simulink model "Totem_Pole_PFC_v1"  (R2024b)
settings: Solver=FixedStepDiscrete  StartTime=0.0  StopTime=0.6  FixedStep=Ts_Power  MaxStep=1e-7  RelTol=1e-4  EnableMultiTasking=on
PreLoadFcn:
  | Totem_Pole_PFC_v1_data
values from neighbouring files (symbols this model uses):
  C_PFC = 2600e-6    (= 0.0026)    [OBC_v1_data.m]    (also in Totem_Pole_PFC_v1_data.m)
  Fnom = 60    [OBC_v1_data.m]    (also in Totem_Pole_PFC_v1_data.m)
  Fr_I = Fnom*2    (= 120)    [OBC_v1_data.m]    (also in Totem_Pole_PFC_v1_data.m)
  Ki_V = 80    [OBC_v1_data.m]    (also in Totem_Pole_PFC_v1_data.m)
  Kp_I = 0.06    [OBC_v1_data.m]    (also in Totem_Pole_PFC_v1_data.m)
  Kp_V = 0.25    [OBC_v1_data.m]    (also in Totem_Pole_PFC_v1_data.m)
  Kr_I = 2.5    [OBC_v1_data.m]    (also in Totem_Pole_PFC_v1_data.m)
  L_PFC = 600e-6    (= 0.0006)    [OBC_v1_data.m]    (also in Totem_Pole_PFC_v1_data.m)
  Limit_V = 100    [OBC_v1_data.m]    (also in Totem_Pole_PFC_v1_data.m)
  RL_PFC = 20e-3    (= 0.02)    [OBC_v1_data.m]    (also in Totem_Pole_PFC_v1_data.m)
  Ro = Vo_nom^2/Po_nom    (= 22.2222222222)    [LLC_Resonant_Converter_v1_data.m]    (also in OBC_v1_data.m; Totem_Pole_PFC_v1_data.m = 22.22)
  Ts_Control = 10e-6    (= 1e-05)    [LLC_Resonant_Converter_v1_data.m]    (also in OBC_v1_data.m; Totem_Pole_PFC_v1_data.m)
  Ts_Power = 50e-9    (= 5e-08)    [LLC_Resonant_Converter_v1_data.m]    (also in OBC_v1_data.m; Totem_Pole_PFC_v1_data.m)
  Vnom_ac = 240    [OBC_v1_data.m]    (also in Totem_Pole_PFC_v1_data.m)
undefined symbols (not defined in the file or in its folder): DiscIntNeverNeededParam
libraries: spsSeriesRLCBranchLib x4, spsDiodeLib x3, spsMeanLib x3, spsCurrentMeasurementLib x2, MyLibrary x2, spsFourierLib x2, simulink x2, spsVoltageMeasurementLib x2, spsACVoltageSourceLib x1, spsIdealSwitchLib x1, spsPowerLib x1, spsTHDLib x1
settings Model: SimulationMode=accelerator  Creator=The MathWorks, Inc.  LastModifiedBy=santh
settings SolverCC: AlgebraicLoopSolver=TrustRegion  SolverResetMethod=Robust
settings DataIOCC: SaveOutput=off  SignalLogging=off  DSMLogging=off  SaveTime=off  ReturnWorkspaceOutputs=off
settings OptimizationCC: LifeSpan=inf
settings DebuggingCC: UnconnectedInputMsg=warning  UnconnectedOutputMsg=warning  UnconnectedLineMsg=warning  SFUnexpectedBacktrackingDiag=warning  SFNoUnconditionalDefaultTransitionDiag=warning  SFExecutionAtInitializationDiag=none  ArithmeticOperatorsInVariantConditions=warning
settings ModelReferenceCC: EnableRefExpFcnMdlSchedulingChecks=on
settings SFSimCC: SimUseLocalCustomCode=off  CustomCodeUndefinedFunction=UseInterfaceOnly
settings RTWCC: RTWUseLocalCustomCode=off  GPUComputeCapability=3.5  DLArmComputeVersion=19.05
settings CodeAppCC: StateflowObjectComments=on
settings GRTTargetCC: TargetLangStandard=C89/C90 (ANSI)
settings ConfigComp: CovMetricSettings=dw  CovSaveCumulativeToWorkspaceVar=on  CovSaveSingleToWorkspaceVar=on  CovExternalEMLEnable=off
settings SimscapeCC: SimscapeNormalizeSystem=off  SimscapeNominalValues={1, 'bar'; 1, 'cm^3/s'; 1, 'bar*kg/s'; 1, 'kJ/kg'; 1, 'kW'; }

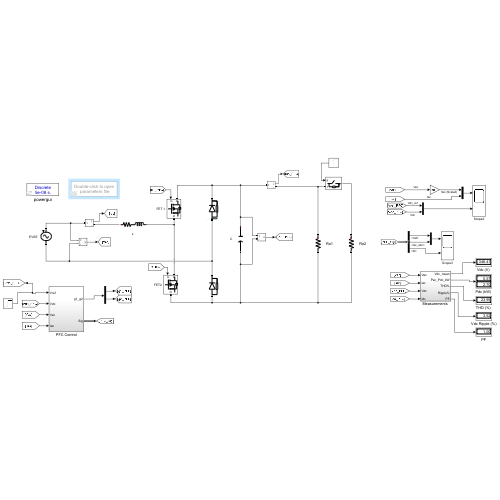
[thumbnail: Simulink's stored preview of the top-level diagram]
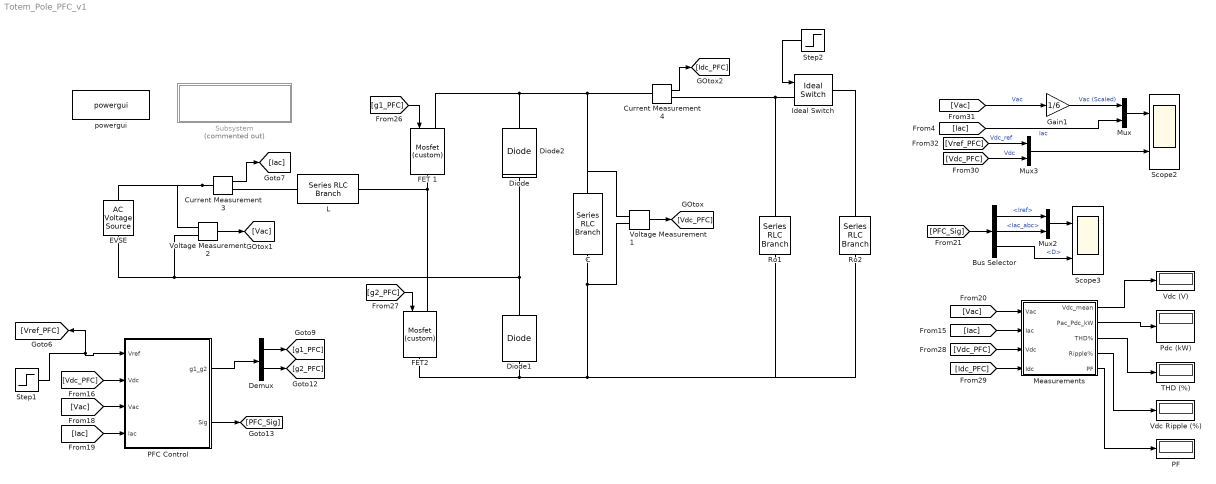
== system Totem_Pole_PFC_v1 ==
  Bus Selector : BusSelector  OutputSignals=Iref,Iac_abc,D
  C : spsSeriesRLCBranchLib/Series RLC Branch  LConnTagsString=__new0  RConnTagsString=__new0  BranchType=C  Resistance=1  Inductance=1e-3  SetiL0=off  InitialCurrent=0  Capacitance=C_PFC  Setx0=on  InitialVoltage=375  Measurements=None
  Current Measurement3 : spsCurrentMeasurementLib/Current Measurement  PhasorSimulation=off  OutputType=Complex  PSBequivalent=0
  Current Measurement4 : spsCurrentMeasurementLib/Current Measurement  PhasorSimulation=off  OutputType=Complex  PSBequivalent=0
  Demux : Demux  Outputs=2
  Diode : spsDiodeLib/Diode  Ron=Ron_Diode  Lon=0  Vf=Vf  IC=0  UseSnubber=0  Rs=1e6  Cs=inf  Measurements=off
  Diode1 : spsDiodeLib/Diode  Ron=Ron_Diode  Lon=0  Vf=Vf  IC=0  UseSnubber=0  Rs=1e6  Cs=inf  Measurements=off
  Diode2 : spsDiodeLib/Diode  Ron=Ron_Diode  Lon=0  Vf=Vf  IC=0  UseSnubber=0  Rs=1e6  Cs=inf  Measurements=off
  EVSE : spsACVoltageSourceLib/AC Voltage Source  Amplitude=Vnom_ac*sqrt(2)  Phase=0  Frequency=Fnom  SampleTime=Ts_Power  Measurements=None  BusType=swing  Pref=10e3  Qref=0  Qmin=-inf  Qmax=+inf
  FET 1 : MyLibrary/Mosfet (custom)  Ron=Ron_FET  Lon=0  Rd=Ron_Diode  Vfd=Vf  IC=0  Rs=1e6  Cs=inf  Measurements=off
  FET2 : MyLibrary/Mosfet (custom)  Ron=Ron_FET  Lon=0  Rd=Ron_Diode  Vfd=Vf  IC=0  Rs=1e6  Cs=inf  Measurements=off
  Gain1 : Gain  Gain=1/6
  Ideal Switch : spsIdealSwitchLib/Ideal Switch  Ron=0.001  Lon=0  IC=0  Rs=1e5  Cs=inf  Measurements=off
  L : spsSeriesRLCBranchLib/Series RLC Branch  LConnTagsString=__new0  RConnTagsString=__new0  BranchType=RL  Resistance=RL_PFC  Inductance=L_PFC  SetiL0=off  InitialCurrent=0  Capacitance=1e-6  Setx0=off  InitialVoltage=0  Measurements=None
  "Measurements " : Subsystem
  Mux : Mux  Inputs=2
  Mux2 : Mux  Inputs=2
  Mux3 : Mux  Inputs=2
  PF : Display
      settings: Format=bank  Decimation=100
  PFC Control : Subsystem
  "Pdc (kW) " : Display
      settings: Format=bank  Decimation=100
  Ro1 : spsSeriesRLCBranchLib/Series RLC Branch  LConnTagsString=__new0  RConnTagsString=__new0  BranchType=R  Resistance=Ro*2  Inductance=200e-6  SetiL0=off  InitialCurrent=0  Capacitance=400e-6  Setx0=off  InitialVoltage=0  Measurements=None
  Ro2 : spsSeriesRLCBranchLib/Series RLC Branch  LConnTagsString=__new0  RConnTagsString=__new0  BranchType=R  Resistance=Ro*2  Inductance=200e-6  SetiL0=off  InitialCurrent=0  Capacitance=400e-6  Setx0=off  InitialVoltage=0  Measurements=None
  Scope2 : Scope  NumInputPorts=2
  Scope3 : Scope  NumInputPorts=2
  Step1 : Step  Time=0.2  Before=350  After=400  SampleTime=Ts_Power
  Step2 : Step  Time=0.4  SampleTime=Ts_Power
  Subsystem : Subsystem  Commented=on
      settings: OpenFcn=edit('Totem_Pole_PFC_v1_data');
      mask Display: disp('Double-click to open\n parameters file');
  "THD (%) " : Display
      settings: Format=bank  Decimation=100
  "Vdc (V) " : Display
      settings: Format=bank  Decimation=100
  Vdc Ripple (%) : Display
      settings: Format=bank  Decimation=100
  Voltage Measurement1 : spsVoltageMeasurementLib/Voltage Measurement  PhasorSimulation=off  OutputType=Complex  PSBequivalent=0
  Voltage Measurement2 : spsVoltageMeasurementLib/Voltage Measurement  PhasorSimulation=off  OutputType=Complex  PSBequivalent=0
  powergui : spspowerguiLib/powergui  Priority=1  SimulationMode=Discrete  SampleTime=Ts_Power  frequency=60  Iterations=50  frequencyindice=0  Pbase=100e6  ErrMax=1e-4  UnitsV=kV  UnitsW=MW  buscounter=0  FunctionMessages=off  echomessages=off  EnableUseOfTLC=off  CurrentSourceSwitches=off  DisableSnubberDevices=off  DisableRonSwitches=off  DisableVfSwitches=off  DisplayEquations=off  AutomaticDiscreteSolvers=off  SolverType=Tustin/Backward Euler (TBE)  Interpol=off  ExternalGateDelay=off  methode=off  Ts=100  x0status=blocks  SPID=on  SwTol=0  HookPort=off  NonlinearTolerance=1e-4  nMaxIteration=100  ContinueOnMaxIteration=off  RestoreLinks=warning  ResistiveCurrentMeasurement=off  Frange=[0:2:500]  Ylog=off  Xlog=on  ShowGrid=off  save=off  variable=ZData  structure=0  ZoomFFT=off  StartTime=0.0  cycles=1  DisplayStyle=1  fundamental=60  FreqAxis=off  MaxFrequency=1000  frequencyindicesteady=1  RmsSteady=1  display=off
  wires:
  Current Measurement4/1 -> [Idc_PFC]
  Voltage Measurement2/1 -> [Vac]
  Voltage Measurement1/1 -> [Vdc_PFC]
  Current Measurement3/1 -> [Iac]
  [Vdc_PFC] -> PFC Control/2(Vdc)
  [Iac] -> PFC Control/4(Iac)
  [Vac] -> PFC Control/3(Vac)
  PFC Control/1(g1_g2) -> Demux/1
  PFC Control/2(Sig) -> [PFC_Sig]
  Step1/1 -> PFC Control/1(Vref), [Vref_PFC]
  Demux/1 -> [g1_PFC]
  Demux/2 -> [g2_PFC]
  [g1_PFC] -> FET 1/1
  [g2_PFC] -> FET2/1
  "Measurements "/4(Ripple%) -> Vdc Ripple (%)/1
  "Measurements "/1(Vdc_mean) -> "Vdc (V) "/1
  [PFC_Sig] -> Bus Selector/1
  Bus Selector/2 -> Mux2/2  "<Iac_abc>"
  "Measurements "/5(PF) -> PF/1
  Bus Selector/3 -> Scope3/2  "<D>"
  Mux2/1 -> Scope3/1
  [Iac] -> Mux/2  "Iac"
  [Idc_PFC] -> "Measurements "/4(Idc)
  [Vref_PFC] -> Mux3/1  "Vdc_ref"
  [Vac] -> "Measurements "/1(Vac)
  [Vac] -> Gain1/1  "Vac"
  Mux3/1 -> Scope2/2
  [Iac] -> "Measurements "/2(Iac)
  Bus Selector/1 -> Mux2/1  "<Iref>"
  [Vdc_PFC] -> Mux3/2  "Vdc"
  "Measurements "/3(THD%) -> "THD (%) "/1
  [Vdc_PFC] -> "Measurements "/3(Vdc)
  "Measurements "/2(Pac_Pdc_kW) -> "Pdc (kW) "/1
  Step2/1 -> Ideal Switch/1
  Gain1/1 -> Mux/1  "Vac (Scaled)"
  Mux/1 -> Scope2/1
  connections:
  Voltage Measurement1/LConn1 -- C/LConn1 -- Current Measurement4/LConn1 -- FET 1/LConn1 -- Diode/RConn1
  L/RConn1 -- FET 1/RConn1 -- FET2/LConn1
  Diode/LConn1 -- Diode1/RConn1 -- Voltage Measurement2/LConn2 -- EVSE/LConn1
  Current Measurement3/LConn1 -- Voltage Measurement2/LConn1 -- EVSE/RConn1
  Current Measurement3/RConn1 -- L/LConn1
  C/RConn1 -- Voltage Measurement1/LConn2 -- Ro2/RConn1 -- Ro1/RConn1 -- FET2/RConn1 -- Diode1/LConn1
  Current Measurement4/RConn1 -- Ideal Switch/LConn1 -- Ro1/LConn1
  Ideal Switch/RConn1 -- Ro2/LConn1

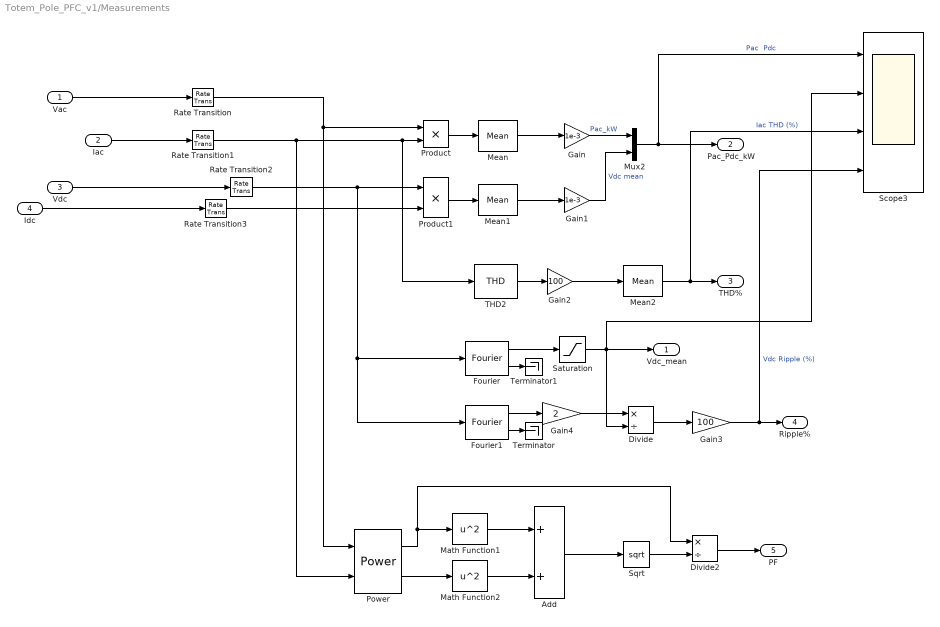
== system Totem_Pole_PFC_v1/Measurements  ==
  Vac : Inport
  Iac : Inport  Port=2
  Vdc : Inport  Port=3
  Idc : Inport  Port=4
  Add : Sum
  Divide : Product  Inputs=*/
  Divide2 : Product  Inputs=*/
  Fourier : spsFourierLib/Fourier  Freq=Fnom  n=0  InInit=[0, 0]  Ts=Ts_Control
  Fourier1 : spsFourierLib/Fourier  Freq=Fnom  n=2  InInit=[0, 0]  Ts=Ts_Control
  Gain : Gain  Gain=1e-3
  Gain1 : Gain  Gain=1e-3
  Gain2 : Gain  Gain=100
  Gain3 : Gain  Gain=100
  Gain4 : Gain  Gain=2
  Math Function1 : Math  Operator=square
  Math Function2 : Math  Operator=square
  Mean : spsMeanLib/Mean  Freq=Fnom  Vinit=0  Ts=Ts_Control
  Mean1 : spsMeanLib/Mean  Freq=Fnom  Vinit=0  Ts=Ts_Control
  Mean2 : spsMeanLib/Mean  Freq=Fnom  Vinit=0  Ts=Ts_Control
  Mux2 : Mux  Inputs=2
  Power : spsPowerLib/Power  Freq=Fnom  Vinit=[1, 0]  Iinit=[1, 0]  Ts=Ts_Control
  Product : Product
  Product1 : Product
  Rate Transition{,1..3} (4 alike) : RateTransition  OutPortSampleTime=Ts_Control
  Saturation : Saturate  UpperLimit=inf  LowerLimit=eps
  Scope3 : Scope  NumInputPorts=4
  Sqrt : Sqrt
  THD2 : spsTHDLib/THD  Freq=Fnom  Ts=Ts_Control
  Terminator : Terminator
  Terminator1 : Terminator
  Vdc_mean : Outport
  Pac_Pdc_kW : Outport  Port=2
  THD% : Outport  Port=3
  Ripple% : Outport  Port=4
  PF : Outport  Port=5
  wires:
  Gain1/1 -> Mux2/2  "Vdc mean"
  Product1/1 -> Mean1/1
  Mean/1 -> Gain/1
  Product/1 -> Mean/1
  Gain/1 -> Mux2/1  "Pac_kW"
  THD2/1 -> Gain2/1
  Mean1/1 -> Gain1/1
  Iac/1 -> Rate Transition1/1
  Mux2/1 -> Scope3/1, Pac_Pdc_kW/1  "Pac  Pdc"
  Gain2/1 -> Mean2/1
  Mean2/1 -> Scope3/3, THD%/1  "Iac THD (%)"
  Fourier/2 -> Terminator1/1
  Fourier/1 -> Saturation/1
  Saturation/1 -> Scope3/2, Vdc_mean/1, Divide/2
  Divide/1 -> Gain3/1
  Fourier1/1 -> Gain4/1
  Gain4/1 -> Divide/1
  Fourier1/2 -> Terminator/1
  Gain3/1 -> Scope3/4, Ripple%/1  "Vdc Ripple (%)"
  Power/1 -> Math Function1/1, Divide2/1
  Power/2 -> Math Function2/1
  Math Function1/1 -> Add/1
  Math Function2/1 -> Add/2
  Add/1 -> Sqrt/1
  Sqrt/1 -> Divide2/2
  Divide2/1 -> PF/1
  Rate Transition1/1 -> Power/2, THD2/1, Product/2
  Vdc/1 -> Rate Transition2/1
  Idc/1 -> Rate Transition3/1
  Rate Transition/1 -> Power/1, Product/1
  Vac/1 -> Rate Transition/1
  Rate Transition2/1 -> Product1/1, Fourier/1, Fourier1/1
  Rate Transition3/1 -> Product1/2

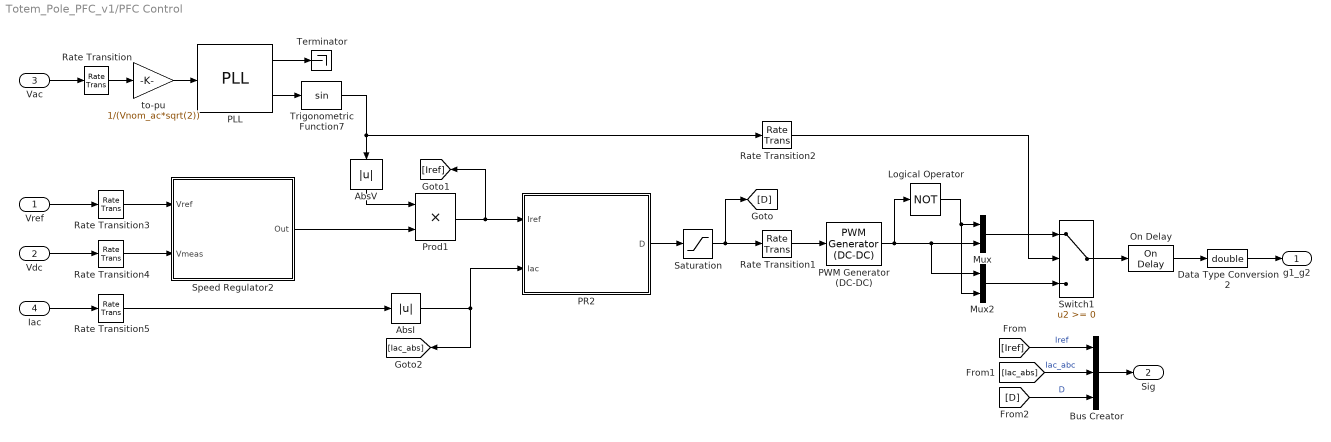
== system Totem_Pole_PFC_v1/PFC Control ==
  Vref : Inport
  Vdc : Inport  Port=2
  Vac : Inport  Port=3
  Iac : Inport  Port=4
  AbsI : Abs  SaturateOnIntegerOverflow=off
  AbsV : Abs  SaturateOnIntegerOverflow=off
  Bus Creator : BusCreator  Inputs=3
  Data Type Conversion2 : DataTypeConversion  OutDataTypeStr=double  SaturateOnIntegerOverflow=off  RndMeth=Floor
  Logical Operator : Logic  Operator=NOT  AllPortsSameDT=off  OutDataTypeStr=float('double')
  Mux : Mux  Inputs=2
  Mux2 : Mux  Inputs=2
  On Delay : spsOnDelayLib/On Delay  DelayType=On delay  delay=DT_PFC  ic=0  Ts=Ts_Power
  PLL : spsPLLLib/PLL  Fmin=0.9*Fnom  Par_Init=[0, Fnom]  ParK=[180, 3200, 1]  TcD=1e-4  MaxRateChangeFreq=12  FilterCutOffFreq=25  Ts=Ts_Control  AGC=on
  PR2 : Subsystem  mask(Current Regulator (Pr)){Kp=Kp_I, Kr=Kr_I, Fr=Fr_I}
      mask prompts: Kp "Proportional gain"; Kr "Resonant gain"; Fr "Resonant frequency (Hz)"
      mask help: This block implements a currentregulator using a PR controller.
      mask Display: disp('Current Regulator\n PR');
  PWM Generator (DC-DC) : spsPWMGeneratorDCDCLib/PWM Generator (DC-DC)  Fsw=Fsw  Ts=Ts_Power
  Prod1 : Product
  Rate Transition{,3..5} (4 alike) : RateTransition  OutPortSampleTime=Ts_Control
  Rate Transition1 : RateTransition  OutPortSampleTime=Ts_Power
  Rate Transition2 : RateTransition  OutPortSampleTime=Ts_Power
  Saturation : Saturate  UpperLimit=1  LowerLimit=0
  Speed Regulator2 : Subsystem  DialogController=POWERSYS.PowerSysDialog  mask(Voltage Regulator){Kp=Kp_V, Ki=Ki_V, Limit_wreg=Limit_V, Init=0, Ts=Ts_Control}
      mask prompts: Kp "Proportional gain (Kp):"; Ki "Integral gain (Ki):"; Limit_wreg "Output limits"; Init "Output initial value:"; Ts "Sample time:"
      mask help: This block implements a voltage regulator using an ant-windup PI controller.
      mask Display: disp('Voltage\nRegulator');
  Switch1 : Switch  SaturateOnIntegerOverflow=off  InputSameDT=off
  Terminator : Terminator
  Trigonometric Function7 : Trigonometry
  to-pu : Gain  Gain=1/(Vnom_ac*sqrt(2))
  g1_g2 : Outport  PortDimensions=2
  Sig : Outport  Port=2
  wires:
  Vdc/1 -> Rate Transition4/1
  Speed Regulator2/1(Out) -> Prod1/2
  Vac/1 -> Rate Transition/1
  AbsV/1 -> Prod1/1
  Vref/1 -> Rate Transition3/1
  Prod1/1 -> PR2/1(Iref), [Iref]
  AbsI/1 -> PR2/2(Iac), [Iac_abs]
  Saturation/1 -> [D], Rate Transition1/1
  Mux/1 -> Switch1/1
  Mux2/1 -> Switch1/3
  Rate Transition1/1 -> PWM Generator (DC-DC)/1
  Bus Creator/1 -> Sig/1
  [Iref] -> Bus Creator/1  "Iref"
  [Iac_abs] -> Bus Creator/2  "Iac_abc"
  [D] -> Bus Creator/3  "D"
  Switch1/1 -> On Delay/1
  PWM Generator (DC-DC)/1 -> Logical Operator/1, Mux2/1, Mux/2
  to-pu/1 -> PLL/1
  PLL/2 -> Trigonometric Function7/1
  Trigonometric Function7/1 -> AbsV/1, Rate Transition2/1
  PLL/1 -> Terminator/1
  PR2/1(D) -> Saturation/1
  Logical Operator/1 -> Mux2/2, Mux/1
  Rate Transition2/1 -> Switch1/2
  Rate Transition/1 -> to-pu/1
  Rate Transition3/1 -> Speed Regulator2/1(Vref)
  Rate Transition4/1 -> Speed Regulator2/2(Vmeas)
  Rate Transition5/1 -> AbsI/1
  Iac/1 -> Rate Transition5/1
  On Delay/1 -> Data Type Conversion2/1
  Data Type Conversion2/1 -> g1_g2/1

== system Totem_Pole_PFC_v1/Subsystem ==

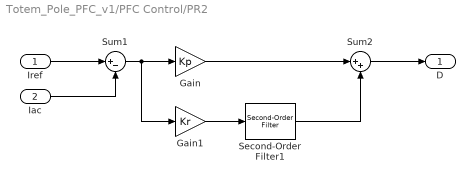
== system Totem_Pole_PFC_v1/PFC Control/PR2 ==
  Iref : Inport
  Iac : Inport  Port=2
  Gain : Gain  Gain=Kp
  Gain1 : Gain  Gain=Kr
  Second-Order Filter1 : spsSecondOrderFilterLib/Second-Order Filter  FilterType=Bandpass  Fo=Fr  Zeta=Zeta_I  Ts=Ts_Control  Initialize=off  Vac_Init="[0,  0,  60]"  Vdc_Init=0  PlotResponse=off  FreqRange=[0, 1000, 0.2]
  Sum1 : Sum  Inputs=|+-
  Sum2 : Sum  Inputs=|++
  D : Outport
  wires:
  Gain1/1 -> Second-Order Filter1/1
  Sum2/1 -> D/1
  Gain/1 -> Sum2/1
  Iac/1 -> Sum1/2
  Iref/1 -> Sum1/1
  Sum1/1 -> Gain1/1, Gain/1
  Second-Order Filter1/1 -> Sum2/2

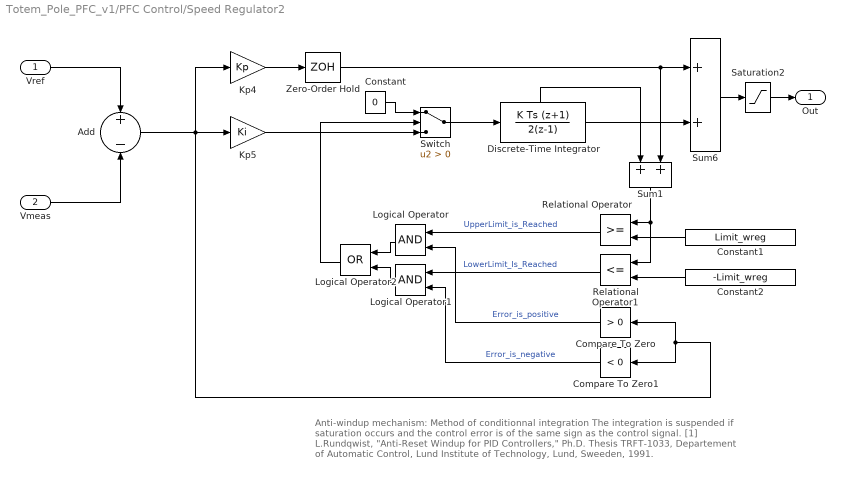
== system Totem_Pole_PFC_v1/PFC Control/Speed Regulator2 ==
  note: Anti-windup mechanism: Method of conditionnal integration
      |
      | The integration is suspended if saturation occurs and the
      | control error is of the same sign as the control signal.
      |
      | [1] L.Rundqwist, "Anti-Reset Windup for PID Controllers," Ph.D. Thesis TRFT-1033,
      | Departement of Automatic Control, Lund Institute of Technology, Lund, Sweeden, 1991.
  Vref : Inport  PortDimensions=1
  Vmeas : Inport  Port=2  PortDimensions=1
  Add : Sum  Inputs=+|-
  Compare To Zero : simulink/Logic and Bit Operations/Compare To Zero  relop=>  OutDataTypeStr=uint8  ZeroCross=off
  Compare To Zero1 : simulink/Logic and Bit Operations/Compare To Zero  relop=<  OutDataTypeStr=uint8  ZeroCross=off
  Constant : Constant  Value=0
  Constant1 : Constant  Value=Limit_wreg
  Constant2 : Constant  Value=-Limit_wreg
  Discrete-Time Integrator : DiscreteIntegrator  IntegratorMethod=Integration: Trapezoidal  InitialCondition=Init  SampleTime=Ts  LimitOutput=on  UpperSaturationLimit=Limit_wreg  LowerSaturationLimit=-Limit_wreg  ShowStatePort=on  ICPrevOutput=DiscIntNeverNeededParam  ICPrevScaledInput=DiscIntNeverNeededParam
  Kp4 : Gain  Gain=Kp  SaturateOnIntegerOverflow=on  SampleTime=Ts  OutDataTypeStr=Inherit: Same as input  ParamDataTypeStr=Inherit: Same as input
  Kp5 : Gain  Gain=Ki  SaturateOnIntegerOverflow=on  SampleTime=Ts  OutDataTypeStr=Inherit: Same as input  ParamDataTypeStr=Inherit: Same as input
  Logical Operator : Logic  AllPortsSameDT=off  OutDataTypeStr=boolean
  Logical Operator1 : Logic  AllPortsSameDT=off  OutDataTypeStr=boolean
  Logical Operator2 : Logic  Operator=OR  AllPortsSameDT=off  OutDataTypeStr=boolean
  Relational Operator : RelationalOperator  OutDataTypeStr=boolean  InputSameDT=off
  Relational Operator1 : RelationalOperator  Operator=<=  OutDataTypeStr=boolean  InputSameDT=off
  Saturation2 : Saturate  UpperLimit=Limit_wreg  LowerLimit=-Limit_wreg  SampleTime=Ts
  Sum1 : Sum  InputSameDT=on  SaturateOnIntegerOverflow=on  SampleTime=Ts  OutDataTypeStr=Inherit: Same as first input
  Sum6 : Sum  InputSameDT=on  SaturateOnIntegerOverflow=on  SampleTime=Ts  OutDataTypeStr=Inherit: Same as first input
  Switch : Switch  Criteria=u2 > Threshold  SaturateOnIntegerOverflow=off  InputSameDT=off
  Zero-Order Hold : ZeroOrderHold  SampleTime=Ts
  Out : Outport  SampleTime=Ts  InitialOutput=0  VectorParamsAs1DForOutWhenUnconnected=off
  wires:
  Kp5/1 -> Switch/3
  Switch/1 -> Discrete-Time Integrator/1
  Saturation2/1 -> Out/1
  Discrete-Time Integrator/1 -> Sum6/2
  Kp4/1 -> Zero-Order Hold/1
  Sum6/1 -> Saturation2/1
  Add/1 -> Compare To Zero/1, Compare To Zero1/1, Kp5/1, Kp4/1
  Compare To Zero1/1 -> Logical Operator1/2  "Error_is_negative"
  Logical Operator1/1 -> Logical Operator2/2
  Logical Operator/1 -> Logical Operator2/1
  Compare To Zero/1 -> Logical Operator/2  "Error_is_positive"
  Constant2/1 -> Relational Operator1/2
  Constant1/1 -> Relational Operator/2
  Relational Operator1/1 -> Logical Operator1/1  "LowerLimit_Is_Reached"
  Relational Operator/1 -> Logical Operator/1  "UpperLimit_is_Reached"
  Logical Operator2/1 -> Switch/2
  Sum1/1 -> Relational Operator/1, Relational Operator1/1
  Discrete-Time Integrator/State -> Sum1/1
  Zero-Order Hold/1 -> Sum6/1, Sum1/2
  Constant/1 -> Switch/1
  Vref/1 -> Add/1
  Vmeas/1 -> Add/2
